simulink model "SB2_mfcn_todo"  (R2024b)
settings: Solver=FixedStepDiscrete  StartTime=0.0  StopTime=1  FixedStep=0.05  RelTol=1e-3
settings Model: Creator=admin  LastModifiedBy=admin

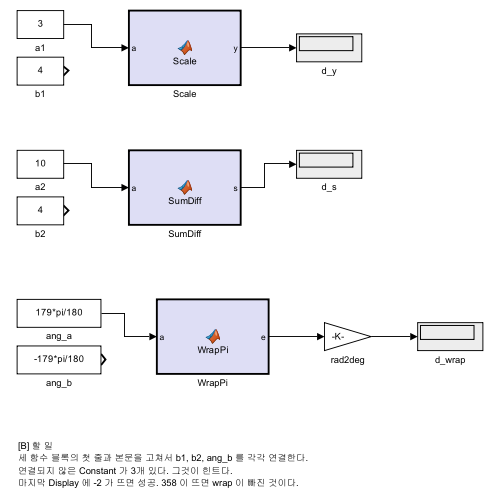
[thumbnail: Simulink's stored preview of the top-level diagram]
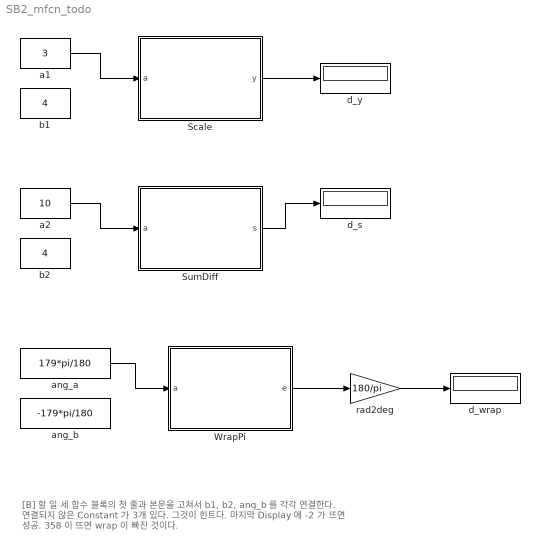
== system SB2_mfcn_todo ==
  note: [B] 할 일
      | 세 함수 블록의 첫 줄과 본문을 고쳐서 b1, b2, ang_b 를 각각 연결한다.
      | 연결되지 않은 Constant 가 3개 있다. 그것이 힌트다.
      | 마지막 Display 에 -2 가 뜨면 성공. 358 이 뜨면 wrap 이 빠진 것이다.
  Scale : MATLAB Function  TreatAsAtomicUnit=on
  SumDiff : MATLAB Function  TreatAsAtomicUnit=on
  WrapPi : MATLAB Function  TreatAsAtomicUnit=on
  a1 : Constant  Value=3
  a2 : Constant  Value=10
  ang_a : Constant  Value=179*pi/180
  ang_b : Constant  Value=-179*pi/180
  b1 : Constant  Value=4
  b2 : Constant  Value=4
  d_s : Display
  d_wrap : Display
  d_y : Display
  rad2deg : Gain  Gain=180/pi
  wires:
  a1/1 -> Scale/1(a)
  Scale/1(y) -> d_y/1
  a2/1 -> SumDiff/1(a)
  SumDiff/1(s) -> d_s/1
  ang_a/1 -> WrapPi/1(a)
  WrapPi/1(e) -> rad2deg/1
  rad2deg/1 -> d_wrap/1

== matlab function SB2_mfcn_todo/Scale ==
  data: a input; y output
function y = Scale(a)
%#codegen
% 할 일: 첫 줄을  function y = Scale(a, b)  로 고치면
%        입력 포트가 2개로 늘어난다. 그 뒤 y = a * b; 로 바꿀 것.
y = a;

== matlab function SB2_mfcn_todo/WrapPi ==
  data: a input; e output
function e = WrapPi(a)
%#codegen
% 할 일: 입력을 (a, b) 두 개로 만들고 아래를 채울 것.
%   d = a - b;
%   e = atan2(sin(d), cos(d));
% Display 에 -2 가 떠야 정답이다 (358 이 아니다).
e = a;

== matlab function SB2_mfcn_todo/SumDiff ==
  data: a input; s output
function s = SumDiff(a)
%#codegen
% 할 일: function [s, d] = SumDiff(a, b) 로 고치고
%        s = a + b;  d = a - b;  를 채울 것.
s = a;
